simulink library "Decoders_Lib"  (Simulink 8.7)
settings: Solver=ode45  StartTime=0.0  StopTime=10.0  RelTol=1e-3
libraries: Computer_Library x17, commutil2 x5
(part 1 of 2)
settings Model: Creator=uzivatel  LastModifiedBy=Jozko Mrkvicka

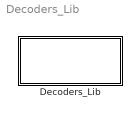
== system Decoders_Lib ==
  Decoders_Lib : Subsystem

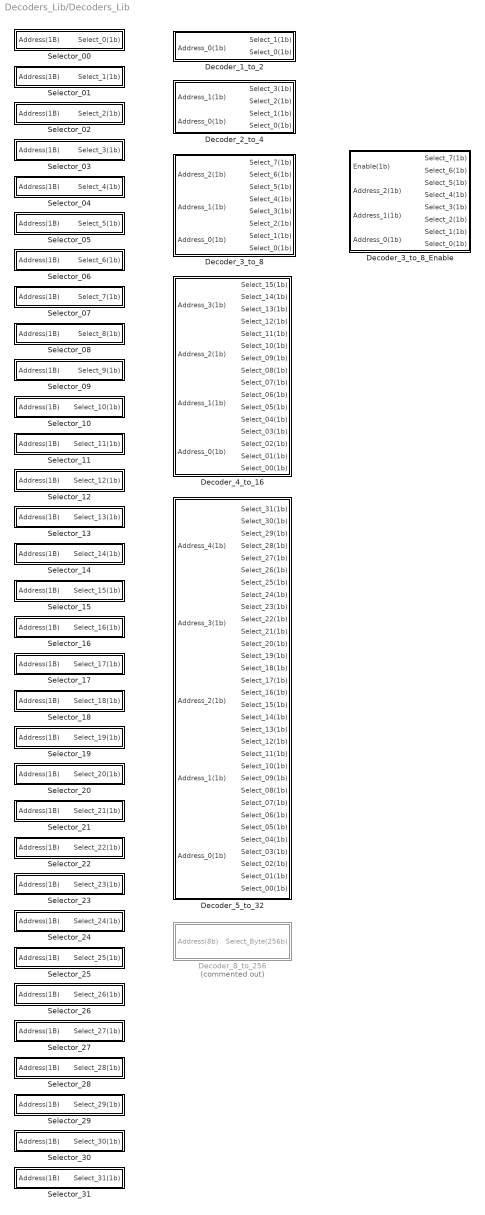
== system Decoders_Lib/Decoders_Lib ==
  Decoder_1_to_2 : Subsystem  TreatAsAtomicUnit=on
  Decoder_2_to_4 : Subsystem  TreatAsAtomicUnit=on
  Decoder_3_to_8 : Subsystem  TreatAsAtomicUnit=on
  Decoder_3_to_8_Enable : Subsystem  TreatAsAtomicUnit=on
  Decoder_4_to_16 : Subsystem  TreatAsAtomicUnit=on
  Decoder_5_to_32 : Subsystem  TreatAsAtomicUnit=on
  Decoder_8_to_256 : Subsystem  Commented=on
  Selector_00 : Subsystem
  Selector_01 : Subsystem
  Selector_02 : Subsystem
  Selector_03 : Subsystem
  Selector_04 : Subsystem
  Selector_05 : Subsystem
  Selector_06 : Subsystem
  Selector_07 : Subsystem
  Selector_08 : Subsystem
  Selector_09 : Subsystem
  Selector_10 : Subsystem
  Selector_11 : Subsystem
  Selector_12 : Subsystem
  Selector_13 : Subsystem
  Selector_14 : Subsystem
  Selector_15 : Subsystem
  Selector_16 : Subsystem
  Selector_17 : Subsystem
  Selector_18 : Subsystem
  Selector_19 : Subsystem
  Selector_20 : Subsystem
  Selector_21 : Subsystem
  Selector_22 : Subsystem
  Selector_23 : Subsystem
  Selector_24 : Subsystem
  Selector_25 : Subsystem
  Selector_26 : Subsystem
  Selector_27 : Subsystem
  Selector_28 : Subsystem
  Selector_29 : Subsystem
  Selector_30 : Subsystem
  Selector_31 : Subsystem

== system Decoders_Lib/Decoders_Lib/Decoder_1_to_2 ==
  Address_0(1b) : Inport
  Logical Operator23 : Logic  Operator=NOT  IconShape=distinctive  AllPortsSameDT=off  OutDataTypeStr=boolean
  Select_1(1b) : Outport
  Select_0(1b) : Outport  Port=2
  wires:
  Logical Operator23/1 -> Select_0(1b)/1
  Address_0(1b)/1 -> Logical Operator23/1, Select_1(1b)/1

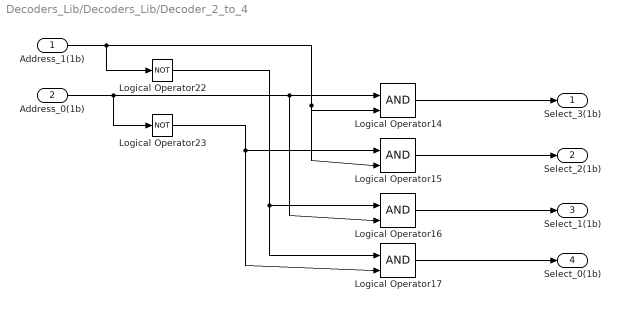
== system Decoders_Lib/Decoders_Lib/Decoder_2_to_4 ==
  Address_1(1b) : Inport
  Address_0(1b) : Inport  Port=2
  Logical Operator{14..17} (4 alike) : Logic  IconShape=distinctive  AllPortsSameDT=off  OutDataTypeStr=boolean
  Logical Operator22 : Logic  Operator=NOT  IconShape=distinctive  AllPortsSameDT=off  OutDataTypeStr=boolean
  Logical Operator23 : Logic  Operator=NOT  IconShape=distinctive  AllPortsSameDT=off  OutDataTypeStr=boolean
  Select_3(1b) : Outport
  Select_2(1b) : Outport  Port=2
  Select_1(1b) : Outport  Port=3
  Select_0(1b) : Outport  Port=4
  wires:
  Address_0(1b)/1 -> Logical Operator23/1, Logical Operator16/2, Logical Operator14/1
  Logical Operator22/1 -> Logical Operator16/1, Logical Operator17/1
  Logical Operator23/1 -> Logical Operator15/1, Logical Operator17/2
  Address_1(1b)/1 -> Logical Operator14/2, Logical Operator15/2, Logical Operator22/1
  Logical Operator17/1 -> Select_0(1b)/1
  Logical Operator16/1 -> Select_1(1b)/1
  Logical Operator15/1 -> Select_2(1b)/1
  Logical Operator14/1 -> Select_3(1b)/1

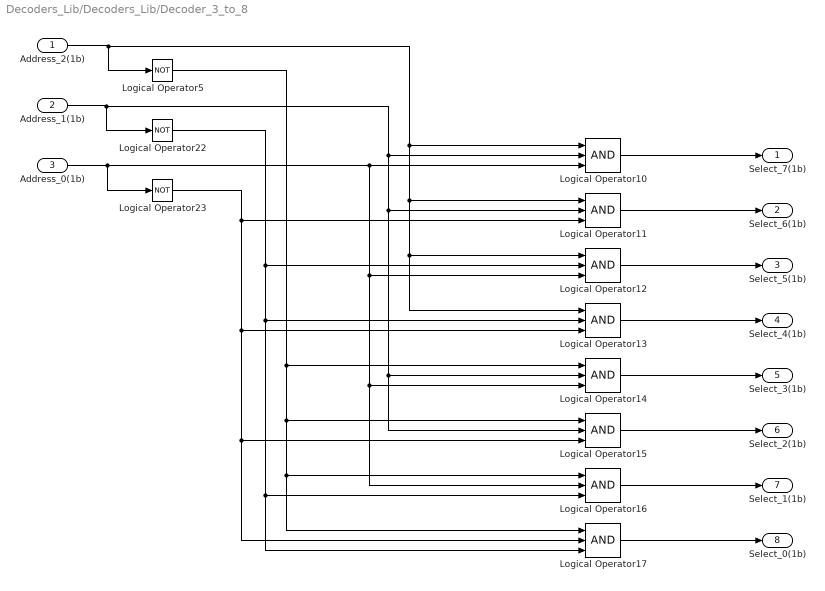
== system Decoders_Lib/Decoders_Lib/Decoder_3_to_8 ==
  "Address_2(1b) " : Inport
  Address_1(1b) : Inport  Port=2
  Address_0(1b) : Inport  Port=3
  Logical Operator{10..17} (8 alike) : Logic  Inputs=3  IconShape=distinctive  AllPortsSameDT=off  OutDataTypeStr=boolean
  Logical Operator22 : Logic  Operator=NOT  IconShape=distinctive  AllPortsSameDT=off  OutDataTypeStr=boolean
  Logical Operator23 : Logic  Operator=NOT  IconShape=distinctive  AllPortsSameDT=off  OutDataTypeStr=boolean
  Logical Operator5 : Logic  Operator=NOT  IconShape=distinctive  AllPortsSameDT=off  OutDataTypeStr=boolean
  Select_7(1b) : Outport
  Select_6(1b) : Outport  Port=2
  Select_5(1b) : Outport  Port=3
  Select_4(1b) : Outport  Port=4
  Select_3(1b) : Outport  Port=5
  Select_2(1b) : Outport  Port=6
  Select_1(1b) : Outport  Port=7
  Select_0(1b) : Outport  Port=8
  wires:
  Address_0(1b)/1 -> Logical Operator10/3, Logical Operator12/3, Logical Operator14/3, Logical Operator16/2, Logical Operator23/1
  Logical Operator22/1 -> Logical Operator12/2, Logical Operator13/2, Logical Operator16/3, Logical Operator17/3
  Logical Operator23/1 -> Logical Operator11/3, Logical Operator13/3, Logical Operator15/3, Logical Operator17/2
  Logical Operator5/1 -> Logical Operator14/1, Logical Operator15/1, Logical Operator16/1, Logical Operator17/1
  Address_1(1b)/1 -> Logical Operator10/2, Logical Operator11/2, Logical Operator14/2, Logical Operator15/2, Logical Operator22/1
  "Address_2(1b) "/1 -> Logical Operator10/1, Logical Operator11/1, Logical Operator12/1, Logical Operator13/1, Logical Operator5/1
  Logical Operator17/1 -> Select_0(1b)/1
  Logical Operator16/1 -> Select_1(1b)/1
  Logical Operator15/1 -> Select_2(1b)/1
  Logical Operator14/1 -> Select_3(1b)/1
  Logical Operator13/1 -> Select_4(1b)/1
  Logical Operator12/1 -> Select_5(1b)/1
  Logical Operator11/1 -> Select_6(1b)/1
  Logical Operator10/1 -> Select_7(1b)/1

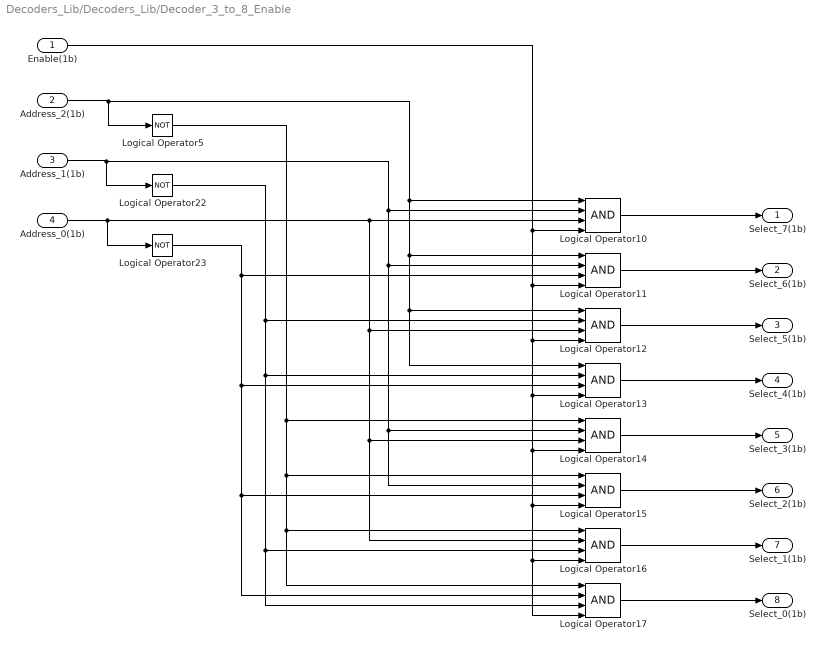
== system Decoders_Lib/Decoders_Lib/Decoder_3_to_8_Enable ==
  Enable(1b) : Inport
  "Address_2(1b) " : Inport  Port=2
  Address_1(1b) : Inport  Port=3
  Address_0(1b) : Inport  Port=4
  Logical Operator{10..17} (8 alike) : Logic  Inputs=4  IconShape=distinctive  AllPortsSameDT=off  OutDataTypeStr=boolean
  Logical Operator22 : Logic  Operator=NOT  IconShape=distinctive  AllPortsSameDT=off  OutDataTypeStr=boolean
  Logical Operator23 : Logic  Operator=NOT  IconShape=distinctive  AllPortsSameDT=off  OutDataTypeStr=boolean
  Logical Operator5 : Logic  Operator=NOT  IconShape=distinctive  AllPortsSameDT=off  OutDataTypeStr=boolean
  Select_7(1b) : Outport
  Select_6(1b) : Outport  Port=2
  Select_5(1b) : Outport  Port=3
  Select_4(1b) : Outport  Port=4
  Select_3(1b) : Outport  Port=5
  Select_2(1b) : Outport  Port=6
  Select_1(1b) : Outport  Port=7
  Select_0(1b) : Outport  Port=8
  wires:
  Address_0(1b)/1 -> Logical Operator10/3, Logical Operator12/3, Logical Operator14/3, Logical Operator16/2, Logical Operator23/1
  Logical Operator22/1 -> Logical Operator12/2, Logical Operator13/2, Logical Operator16/3, Logical Operator17/3
  Logical Operator23/1 -> Logical Operator11/3, Logical Operator13/3, Logical Operator15/3, Logical Operator17/2
  Logical Operator5/1 -> Logical Operator14/1, Logical Operator15/1, Logical Operator16/1, Logical Operator17/1
  Address_1(1b)/1 -> Logical Operator11/2, Logical Operator14/2, Logical Operator15/2, Logical Operator10/2, Logical Operator22/1
  "Address_2(1b) "/1 -> Logical Operator11/1, Logical Operator12/1, Logical Operator13/1, Logical Operator10/1, Logical Operator5/1
  Logical Operator17/1 -> Select_0(1b)/1
  Logical Operator16/1 -> Select_1(1b)/1
  Logical Operator15/1 -> Select_2(1b)/1
  Logical Operator14/1 -> Select_3(1b)/1
  Logical Operator13/1 -> Select_4(1b)/1
  Logical Operator12/1 -> Select_5(1b)/1
  Logical Operator11/1 -> Select_6(1b)/1
  Logical Operator10/1 -> Select_7(1b)/1
  Enable(1b)/1 -> Logical Operator10/4, Logical Operator11/4, Logical Operator12/4, Logical Operator14/4, Logical Operator15/4, Logical Operator16/4, Logical Operator17/4, Logical Operator13/4

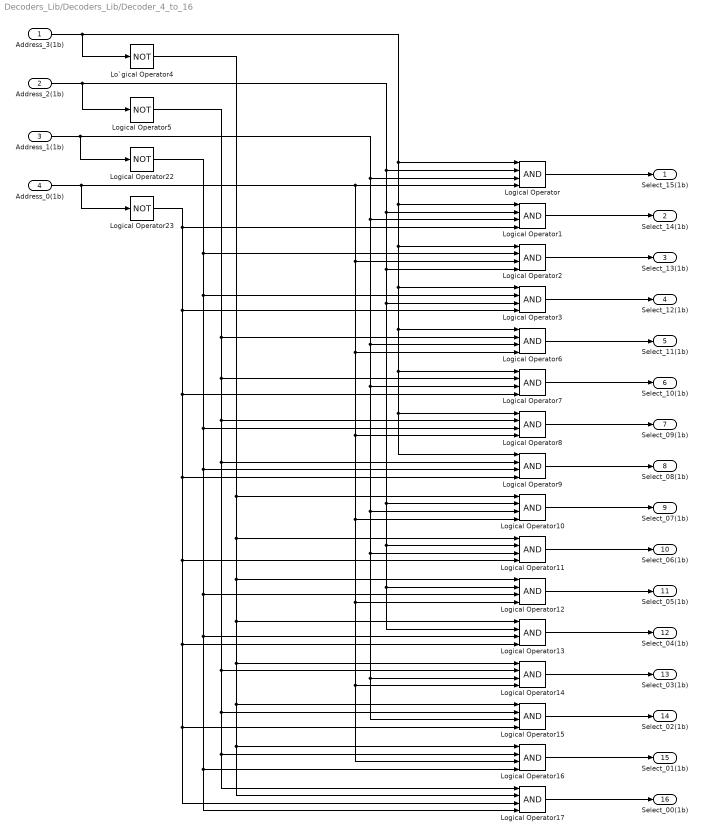
== system Decoders_Lib/Decoders_Lib/Decoder_4_to_16 ==
  Address_3(1b) : Inport
  "Address_2(1b) " : Inport  Port=2
  Address_1(1b) : Inport  Port=3
  Address_0(1b) : Inport  Port=4
  Lo`gical Operator4 : Logic  Operator=NOT  IconShape=distinctive  AllPortsSameDT=off  OutDataTypeStr=boolean
  Logical Operator{,1..3,6..17} (16 alike) : Logic  Inputs=4  IconShape=distinctive  AllPortsSameDT=off  OutDataTypeStr=boolean
  Logical Operator22 : Logic  Operator=NOT  IconShape=distinctive  AllPortsSameDT=off  OutDataTypeStr=boolean
  Logical Operator23 : Logic  Operator=NOT  IconShape=distinctive  AllPortsSameDT=off  OutDataTypeStr=boolean
  Logical Operator5 : Logic  Operator=NOT  IconShape=distinctive  AllPortsSameDT=off  OutDataTypeStr=boolean
  Select_15(1b) : Outport
  Select_14(1b) : Outport  Port=2
  Select_13(1b) : Outport  Port=3
  Select_12(1b) : Outport  Port=4
  Select_11(1b) : Outport  Port=5
  Select_10(1b) : Outport  Port=6
  Select_09(1b) : Outport  Port=7
  Select_08(1b) : Outport  Port=8
  Select_07(1b) : Outport  Port=9
  Select_06(1b) : Outport  Port=10
  Select_05(1b) : Outport  Port=11
  Select_04(1b) : Outport  Port=12
  Select_03(1b) : Outport  Port=13
  Select_02(1b) : Outport  Port=14
  Select_01(1b) : Outport  Port=15
  Select_00(1b) : Outport  Port=16
  wires:
  Logical Operator22/1 -> Logical Operator2/2, Logical Operator3/2, Logical Operator8/3, Logical Operator9/3, Logical Operator12/3, Logical Operator13/3, Logical Operator16/4, Logical Operator17/4
  Address_0(1b)/1 -> Logical Operator/4, Logical Operator2/3, Logical Operator6/4, Logical Operator8/4, Logical Operator10/4, Logical Operator12/4, Logical Operator14/4, Logical Operator16/3, Logical Operator23/1
  Logical Operator23/1 -> Logical Operator1/4, Logical Operator3/4, Logical Operator7/4, Logical Operator9/4, Logical Operator11/4, Logical Operator13/4, Logical Operator15/4, Logical Operator17/3
  Logical Operator5/1 -> Logical Operator6/2, Logical Operator7/2, Logical Operator8/2, Logical Operator9/2, Logical Operator14/2, Logical Operator15/2, Logical Operator16/2, Logical Operator17/1
  Address_3(1b)/1 -> Lo`gical Operator4/1, Logical Operator2/1, Logical Operator3/1, Logical Operator6/1, Logical Operator7/1, Logical Operator8/1, Logical Operator9/1, Logical Operator1/1, Logical Operator/1
  Address_1(1b)/1 -> Logical Operator22/1, Logical Operator/3, Logical Operator1/3, Logical Operator6/3, Logical Operator7/3, Logical Operator10/3, Logical Operator11/3, Logical Operator14/3, Logical Operator15/3
  "Address_2(1b) "/1 -> Logical Operator/2, Logical Operator1/2, Logical Operator2/4, Logical Operator3/3, Logical Operator10/2, Logical Operator11/2, Logical Operator12/2, Logical Operator13/2, Logical Operator5/1
  Lo`gical Operator4/1 -> Logical Operator10/1, Logical Operator11/1, Logical Operator12/1, Logical Operator13/1, Logical Operator14/1, Logical Operator15/1, Logical Operator16/1, Logical Operator17/2
  Logical Operator17/1 -> Select_00(1b)/1
  Logical Operator16/1 -> Select_01(1b)/1
  Logical Operator15/1 -> Select_02(1b)/1
  Logical Operator14/1 -> Select_03(1b)/1
  Logical Operator13/1 -> Select_04(1b)/1
  Logical Operator12/1 -> Select_05(1b)/1
  Logical Operator11/1 -> Select_06(1b)/1
  Logical Operator10/1 -> Select_07(1b)/1
  Logical Operator9/1 -> Select_08(1b)/1
  Logical Operator8/1 -> Select_09(1b)/1
  Logical Operator7/1 -> Select_10(1b)/1
  Logical Operator6/1 -> Select_11(1b)/1
  Logical Operator1/1 -> Select_14(1b)/1
  Logical Operator2/1 -> Select_13(1b)/1
  Logical Operator3/1 -> Select_12(1b)/1
  Logical Operator/1 -> Select_15(1b)/1

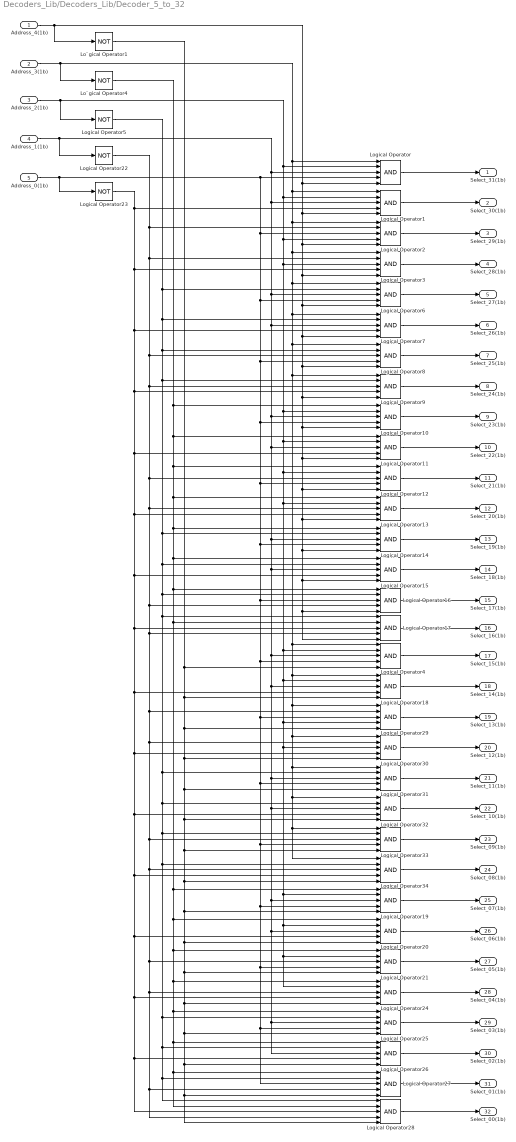
== system Decoders_Lib/Decoders_Lib/Decoder_5_to_32 ==
  Address_4(1b) : Inport
  Address_3(1b) : Inport  Port=2
  "Address_2(1b) " : Inport  Port=3
  Address_1(1b) : Inport  Port=4
  Address_0(1b) : Inport  Port=5
  Lo`gical Operator1 : Logic  Operator=NOT  IconShape=distinctive  AllPortsSameDT=off  OutDataTypeStr=boolean
  Lo`gical Operator4 : Logic  Operator=NOT  IconShape=distinctive  AllPortsSameDT=off  OutDataTypeStr=boolean
  Logical Operator{,1..4,6..21,24..34} (32 alike) : Logic  Inputs=5  IconShape=distinctive  AllPortsSameDT=off  OutDataTypeStr=boolean
  Logical Operator22 : Logic  Operator=NOT  IconShape=distinctive  AllPortsSameDT=off  OutDataTypeStr=boolean
  Logical Operator23 : Logic  Operator=NOT  IconShape=distinctive  AllPortsSameDT=off  OutDataTypeStr=boolean
  Logical Operator5 : Logic  Operator=NOT  IconShape=distinctive  AllPortsSameDT=off  OutDataTypeStr=boolean
  Select_31(1b) : Outport
  Select_30(1b) : Outport  Port=2
  Select_29(1b) : Outport  Port=3
  Select_28(1b) : Outport  Port=4
  Select_27(1b) : Outport  Port=5
  Select_26(1b) : Outport  Port=6
  Select_25(1b) : Outport  Port=7
  Select_24(1b) : Outport  Port=8
  Select_23(1b) : Outport  Port=9
  Select_22(1b) : Outport  Port=10
  Select_21(1b) : Outport  Port=11
  Select_20(1b) : Outport  Port=12
  Select_19(1b) : Outport  Port=13
  Select_18(1b) : Outport  Port=14
  Select_17(1b) : Outport  Port=15
  Select_16(1b) : Outport  Port=16
  Select_15(1b) : Outport  Port=17
  Select_14(1b) : Outport  Port=18
  Select_13(1b) : Outport  Port=19
  Select_12(1b) : Outport  Port=20
  Select_11(1b) : Outport  Port=21
  Select_10(1b) : Outport  Port=22
  Select_09(1b) : Outport  Port=23
  Select_08(1b) : Outport  Port=24
  Select_07(1b) : Outport  Port=25
  Select_06(1b) : Outport  Port=26
  Select_05(1b) : Outport  Port=27
  Select_04(1b) : Outport  Port=28
  Select_03(1b) : Outport  Port=29
  Select_02(1b) : Outport  Port=30
  Select_01(1b) : Outport  Port=31
  Select_00(1b) : Outport  Port=32
  wires:
  Logical Operator17/1 -> Select_16(1b)/1
  Logical Operator16/1 -> Select_17(1b)/1
  Logical Operator15/1 -> Select_18(1b)/1
  Logical Operator14/1 -> Select_19(1b)/1
  Logical Operator13/1 -> Select_20(1b)/1
  Logical Operator12/1 -> Select_21(1b)/1
  Logical Operator11/1 -> Select_22(1b)/1
  Logical Operator10/1 -> Select_23(1b)/1
  Logical Operator9/1 -> Select_24(1b)/1
  Logical Operator8/1 -> Select_25(1b)/1
  Logical Operator7/1 -> Select_26(1b)/1
  Logical Operator6/1 -> Select_27(1b)/1
  Logical Operator1/1 -> Select_30(1b)/1
  Logical Operator2/1 -> Select_29(1b)/1
  Logical Operator3/1 -> Select_28(1b)/1
  Logical Operator/1 -> Select_31(1b)/1
  Logical Operator22/1 -> Logical Operator8/3, Logical Operator9/3, Logical Operator12/3, Logical Operator13/3, Logical Operator16/4, Logical Operator29/2, Logical Operator30/2, Logical Operator33/3, Logical Operator34/3, Logical Operator21/3, Logical Operator24/3, Logical Operator27/4, Logical Operator28/4, Logical Operator17/4, Logical Operator3/2, Logical Operator2/2
  Address_0(1b)/1 -> Logical Operator/4, Logical Operator2/3, Logical Operator6/4, Logical Operator8/4, Logical Operator10/4, Logical Operator12/4, Logical Operator14/4, Logical Operator16/3, Logical Operator4/4, Logical Operator29/3, Logical Operator31/4, Logical Operator33/4, Logical Operator19/4, Logical Operator21/4, Logical Operator25/4, Logical Operator27/3, Logical Operator23/1
  Logical Operator23/1 -> Logical Operator1/4, Logical Operator3/4, Logical Operator7/4, Logical Operator9/4, Logical Operator11/4, Logical Operator13/4, Logical Operator15/4, Logical Operator18/4, Logical Operator30/4, Logical Operator32/4, Logical Operator34/4, Logical Operator20/4, Logical Operator24/4, Logical Operator26/4, Logical Operator28/3, Logical Operator17/3
  Logical Operator5/1 -> Logical Operator31/2, Logical Operator32/2, Logical Operator33/2, Logical Operator34/2, Logical Operator25/2, Logical Operator26/2, Logical Operator27/2, Logical Operator28/1, Logical Operator17/1, Logical Operator16/2, Logical Operator15/2, Logical Operator14/2, Logical Operator9/2, Logical Operator8/2, Logical Operator7/2, Logical Operator6/2
  Address_3(1b)/1 -> Lo`gical Operator4/1, Logical Operator2/1, Logical Operator3/1, Logical Operator6/1, Logical Operator7/1, Logical Operator8/1, Logical Operator4/1, Logical Operator18/1, Logical Operator29/1, Logical Operator30/1, Logical Operator31/1, Logical Operator32/1, Logical Operator33/1, Logical Operator34/1, Logical Operator9/1, Logical Operator1/1, Logical Operator/1
  Address_1(1b)/1 -> Logical Operator22/1, Logical Operator1/3, Logical Operator6/3, Logical Operator7/3, Logical Operator10/3, Logical Operator11/3, Logical Operator14/3, Logical Operator4/3, Logical Operator18/3, Logical Operator31/3, Logical Operator32/3, Logical Operator19/3, Logical Operator20/3, Logical Operator25/3, Logical Operator26/3, Logical Operator15/3, Logical Operator/3
  "Address_2(1b) "/1 -> Logical Operator2/4, Logical Operator3/3, Logical Operator4/2, Logical Operator18/2, Logical Operator29/4, Logical Operator30/3, Logical Operator19/2, Logical Operator20/2, Logical Operator21/2, Logical Operator24/2, Logical Operator13/2, Logical Operator12/2, Logical Operator11/2, Logical Operator10/2, Logical Operator1/2, Logical Operator/2, Logical Operator5/1
  Lo`gical Operator4/1 -> Logical Operator19/1, Logical Operator20/1, Logical Operator21/1, Logical Operator24/1, Logical Operator25/1, Logical Operator26/1, Logical Operator27/1, Logical Operator28/2, Logical Operator17/2, Logical Operator16/1, Logical Operator15/1, Logical Operator14/1, Logical Operator13/1, Logical Operator12/1, Logical Operator11/1, Logical Operator10/1
  Logical Operator28/1 -> Select_00(1b)/1
  Logical Operator27/1 -> Select_01(1b)/1
  Logical Operator26/1 -> Select_02(1b)/1
  Logical Operator25/1 -> Select_03(1b)/1
  Logical Operator24/1 -> Select_04(1b)/1
  Logical Operator21/1 -> Select_05(1b)/1
  Logical Operator20/1 -> Select_06(1b)/1
  Logical Operator19/1 -> Select_07(1b)/1
  Logical Operator34/1 -> Select_08(1b)/1
  Logical Operator33/1 -> Select_09(1b)/1
  Logical Operator32/1 -> Select_10(1b)/1
  Logical Operator31/1 -> Select_11(1b)/1
  Logical Operator18/1 -> Select_14(1b)/1
  Logical Operator29/1 -> Select_13(1b)/1
  Logical Operator30/1 -> Select_12(1b)/1
  Logical Operator4/1 -> Select_15(1b)/1
  Lo`gical Operator1/1 -> Logical Operator4/5, Logical Operator18/5, Logical Operator29/5, Logical Operator30/5, Logical Operator31/5, Logical Operator32/5, Logical Operator33/5, Logical Operator34/5, Logical Operator19/5, Logical Operator20/5, Logical Operator21/5, Logical Operator24/5, Logical Operator25/5, Logical Operator26/5, Logical Operator27/5, Logical Operator28/5
  Address_4(1b)/1 -> Lo`gical Operator1/1, Logical Operator/5, Logical Operator1/5, Logical Operator2/5, Logical Operator3/5, Logical Operator6/5, Logical Operator7/5, Logical Operator8/5, Logical Operator9/5, Logical Operator10/5, Logical Operator11/5, Logical Operator12/5, Logical Operator13/5, Logical Operator14/5, Logical Operator15/5, Logical Operator16/5, Logical Operator17/5

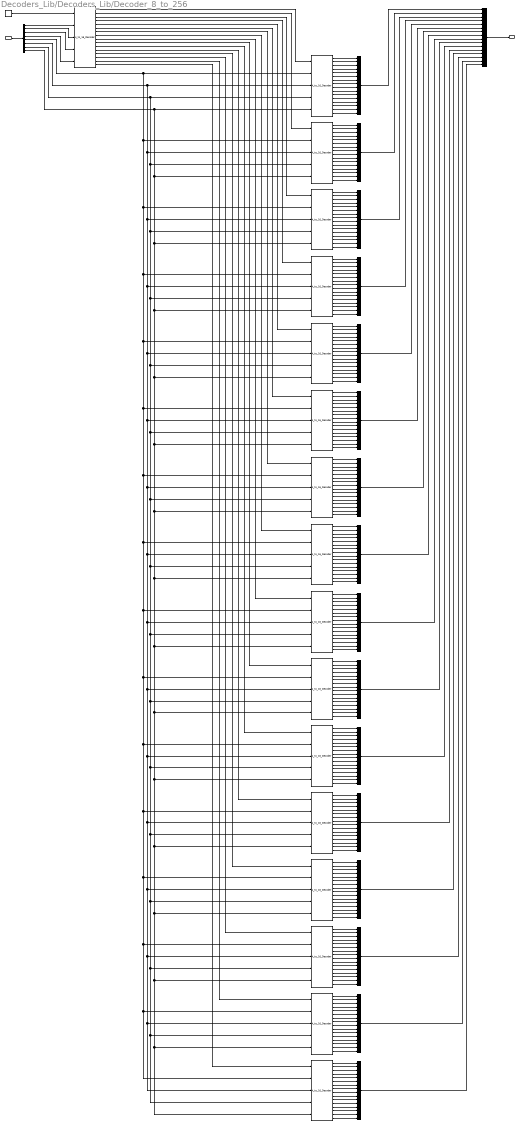
== system Decoders_Lib/Decoders_Lib/Decoder_8_to_256 ==
  Address(8b) : Inport
  4_to_16_Decoder{,1..16} (17 alike) : Computer_Library/4_to_16_Decoder
  Demux : Demux  Outputs=8
  Enable : Constant
  Mux{,1..16} (17 alike) : Mux  Inputs=16
  Select_Byte(256b) : Outport
  wires:
  Mux/1 -> Select_Byte(256b)/1
  Address(8b)/1 -> Demux/1
  Mux2/1 -> Mux/2
  Mux3/1 -> Mux/3
  Mux4/1 -> Mux/4
  Mux5/1 -> Mux/5
  Mux6/1 -> Mux/6
  Mux7/1 -> Mux/7
  Mux8/1 -> Mux/8
  Mux9/1 -> Mux/9
  Mux10/1 -> Mux/10
  Mux11/1 -> Mux/11
  Mux12/1 -> Mux/12
  Mux13/1 -> Mux/13
  Mux14/1 -> Mux/14
  Mux15/1 -> Mux/15
  Mux16/1 -> Mux/16
  Mux1/1 -> Mux/1
  4_to_16_Decoder16/16 -> Mux16/16
  4_to_16_Decoder16/15 -> Mux16/15
  4_to_16_Decoder16/14 -> Mux16/14
  4_to_16_Decoder16/13 -> Mux16/13
  4_to_16_Decoder16/12 -> Mux16/12
  4_to_16_Decoder16/11 -> Mux16/11
  4_to_16_Decoder16/10 -> Mux16/10
  4_to_16_Decoder16/9 -> Mux16/9
  4_to_16_Decoder16/8 -> Mux16/8
  4_to_16_Decoder16/7 -> Mux16/7
  4_to_16_Decoder16/6 -> Mux16/6
  4_to_16_Decoder16/5 -> Mux16/5
  4_to_16_Decoder16/4 -> Mux16/4
  4_to_16_Decoder16/3 -> Mux16/3
  4_to_16_Decoder16/2 -> Mux16/2
  4_to_16_Decoder16/1 -> Mux16/1
  4_to_16_Decoder15/16 -> Mux15/16
  4_to_16_Decoder15/15 -> Mux15/15
  4_to_16_Decoder15/14 -> Mux15/14
  4_to_16_Decoder15/13 -> Mux15/13
  4_to_16_Decoder15/12 -> Mux15/12
  4_to_16_Decoder15/11 -> Mux15/11
  4_to_16_Decoder15/10 -> Mux15/10
  4_to_16_Decoder15/9 -> Mux15/9
  4_to_16_Decoder15/8 -> Mux15/8
  4_to_16_Decoder15/7 -> Mux15/7
  4_to_16_Decoder15/6 -> Mux15/6
  4_to_16_Decoder15/5 -> Mux15/5
  4_to_16_Decoder15/4 -> Mux15/4
  4_to_16_Decoder15/3 -> Mux15/3
  4_to_16_Decoder15/2 -> Mux15/2
  4_to_16_Decoder15/1 -> Mux15/1
  4_to_16_Decoder14/16 -> Mux14/16
  4_to_16_Decoder14/15 -> Mux14/15
  4_to_16_Decoder14/14 -> Mux14/14
  4_to_16_Decoder14/13 -> Mux14/13
  4_to_16_Decoder14/12 -> Mux14/12
  4_to_16_Decoder14/11 -> Mux14/11
  4_to_16_Decoder14/10 -> Mux14/10
  4_to_16_Decoder14/9 -> Mux14/9
  4_to_16_Decoder14/8 -> Mux14/8
  4_to_16_Decoder14/7 -> Mux14/7
  4_to_16_Decoder14/6 -> Mux14/6
  4_to_16_Decoder14/5 -> Mux14/5
  4_to_16_Decoder14/4 -> Mux14/4
  4_to_16_Decoder14/3 -> Mux14/3
  4_to_16_Decoder14/2 -> Mux14/2
  4_to_16_Decoder14/1 -> Mux14/1
  4_to_16_Decoder13/16 -> Mux13/16
  4_to_16_Decoder13/15 -> Mux13/15
  4_to_16_Decoder13/14 -> Mux13/14
  4_to_16_Decoder13/13 -> Mux13/13
  4_to_16_Decoder13/12 -> Mux13/12
  4_to_16_Decoder13/11 -> Mux13/11
  4_to_16_Decoder13/10 -> Mux13/10
  4_to_16_Decoder13/9 -> Mux13/9
  4_to_16_Decoder13/8 -> Mux13/8
  4_to_16_Decoder13/7 -> Mux13/7
  4_to_16_Decoder13/6 -> Mux13/6
  4_to_16_Decoder13/5 -> Mux13/5
  4_to_16_Decoder13/4 -> Mux13/4
  4_to_16_Decoder13/3 -> Mux13/3
  4_to_16_Decoder13/2 -> Mux13/2
  4_to_16_Decoder13/1 -> Mux13/1
  4_to_16_Decoder12/16 -> Mux12/16
  4_to_16_Decoder12/15 -> Mux12/15
  4_to_16_Decoder12/14 -> Mux12/14
  4_to_16_Decoder12/13 -> Mux12/13
  4_to_16_Decoder12/12 -> Mux12/12
  4_to_16_Decoder12/11 -> Mux12/11
  4_to_16_Decoder12/10 -> Mux12/10
  4_to_16_Decoder12/9 -> Mux12/9
  4_to_16_Decoder12/8 -> Mux12/8
  4_to_16_Decoder12/7 -> Mux12/7
  4_to_16_Decoder12/6 -> Mux12/6
  4_to_16_Decoder12/5 -> Mux12/5
  4_to_16_Decoder12/4 -> Mux12/4
  4_to_16_Decoder12/3 -> Mux12/3
  4_to_16_Decoder12/2 -> Mux12/2
  4_to_16_Decoder12/1 -> Mux12/1
  4_to_16_Decoder11/16 -> Mux11/16
  4_to_16_Decoder11/15 -> Mux11/15
  4_to_16_Decoder11/14 -> Mux11/14
  4_to_16_Decoder11/13 -> Mux11/13
  4_to_16_Decoder11/12 -> Mux11/12
  4_to_16_Decoder11/11 -> Mux11/11
  4_to_16_Decoder11/10 -> Mux11/10
  4_to_16_Decoder11/9 -> Mux11/9
  4_to_16_Decoder11/8 -> Mux11/8
  4_to_16_Decoder11/7 -> Mux11/7
  4_to_16_Decoder11/6 -> Mux11/6
  4_to_16_Decoder11/5 -> Mux11/5
  4_to_16_Decoder11/4 -> Mux11/4
  4_to_16_Decoder11/3 -> Mux11/3
  4_to_16_Decoder11/2 -> Mux11/2
  4_to_16_Decoder11/1 -> Mux11/1
  4_to_16_Decoder10/16 -> Mux10/16
  4_to_16_Decoder10/15 -> Mux10/15
  4_to_16_Decoder10/14 -> Mux10/14
  4_to_16_Decoder10/13 -> Mux10/13
  4_to_16_Decoder10/12 -> Mux10/12
  4_to_16_Decoder10/11 -> Mux10/11
  4_to_16_Decoder10/10 -> Mux10/10
  4_to_16_Decoder10/9 -> Mux10/9
  4_to_16_Decoder10/8 -> Mux10/8
  4_to_16_Decoder10/7 -> Mux10/7
  4_to_16_Decoder10/6 -> Mux10/6
  4_to_16_Decoder10/5 -> Mux10/5
  4_to_16_Decoder10/4 -> Mux10/4
  4_to_16_Decoder10/3 -> Mux10/3
  4_to_16_Decoder10/2 -> Mux10/2
  4_to_16_Decoder10/1 -> Mux10/1
  4_to_16_Decoder9/16 -> Mux9/16
  4_to_16_Decoder9/15 -> Mux9/15
  4_to_16_Decoder9/14 -> Mux9/14
  4_to_16_Decoder9/13 -> Mux9/13
  4_to_16_Decoder9/12 -> Mux9/12
  4_to_16_Decoder9/11 -> Mux9/11
  4_to_16_Decoder9/10 -> Mux9/10
  4_to_16_Decoder9/9 -> Mux9/9
  4_to_16_Decoder9/8 -> Mux9/8
  4_to_16_Decoder9/7 -> Mux9/7
  4_to_16_Decoder9/6 -> Mux9/6
  4_to_16_Decoder9/5 -> Mux9/5
  4_to_16_Decoder9/4 -> Mux9/4
  4_to_16_Decoder9/3 -> Mux9/3
  4_to_16_Decoder9/2 -> Mux9/2
  4_to_16_Decoder9/1 -> Mux9/1
  4_to_16_Decoder8/16 -> Mux8/16
  4_to_16_Decoder8/15 -> Mux8/15
  4_to_16_Decoder8/14 -> Mux8/14
  4_to_16_Decoder8/13 -> Mux8/13
  4_to_16_Decoder8/12 -> Mux8/12
  4_to_16_Decoder8/11 -> Mux8/11
  4_to_16_Decoder8/10 -> Mux8/10
  4_to_16_Decoder8/9 -> Mux8/9
  4_to_16_Decoder8/8 -> Mux8/8
  4_to_16_Decoder8/7 -> Mux8/7
  4_to_16_Decoder8/6 -> Mux8/6
  4_to_16_Decoder8/5 -> Mux8/5
  4_to_16_Decoder8/4 -> Mux8/4
  4_to_16_Decoder8/3 -> Mux8/3
  4_to_16_Decoder8/2 -> Mux8/2
  4_to_16_Decoder8/1 -> Mux8/1
  4_to_16_Decoder7/16 -> Mux7/16
  4_to_16_Decoder7/15 -> Mux7/15
  4_to_16_Decoder7/14 -> Mux7/14
  4_to_16_Decoder7/13 -> Mux7/13
  4_to_16_Decoder7/12 -> Mux7/12
  4_to_16_Decoder7/11 -> Mux7/11
  4_to_16_Decoder7/10 -> Mux7/10
  4_to_16_Decoder7/9 -> Mux7/9
  4_to_16_Decoder7/8 -> Mux7/8
  4_to_16_Decoder7/7 -> Mux7/7
  4_to_16_Decoder7/6 -> Mux7/6
  4_to_16_Decoder7/5 -> Mux7/5
  4_to_16_Decoder7/4 -> Mux7/4
  4_to_16_Decoder7/3 -> Mux7/3
  4_to_16_Decoder7/2 -> Mux7/2
  4_to_16_Decoder7/1 -> Mux7/1
  4_to_16_Decoder6/16 -> Mux6/16
  4_to_16_Decoder6/15 -> Mux6/15
  4_to_16_Decoder6/14 -> Mux6/14
  4_to_16_Decoder6/13 -> Mux6/13
  4_to_16_Decoder6/12 -> Mux6/12
  4_to_16_Decoder6/11 -> Mux6/11
  4_to_16_Decoder6/10 -> Mux6/10
  4_to_16_Decoder6/9 -> Mux6/9
  4_to_16_Decoder6/8 -> Mux6/8
  4_to_16_Decoder6/7 -> Mux6/7
  4_to_16_Decoder6/6 -> Mux6/6
  4_to_16_Decoder6/5 -> Mux6/5
  4_to_16_Decoder6/4 -> Mux6/4
  4_to_16_Decoder6/3 -> Mux6/3
  4_to_16_Decoder6/2 -> Mux6/2
  4_to_16_Decoder6/1 -> Mux6/1
  4_to_16_Decoder5/16 -> Mux5/16
  4_to_16_Decoder5/15 -> Mux5/15
  4_to_16_Decoder5/14 -> Mux5/14
  4_to_16_Decoder5/13 -> Mux5/13
  4_to_16_Decoder5/12 -> Mux5/12
  4_to_16_Decoder5/11 -> Mux5/11
  4_to_16_Decoder5/10 -> Mux5/10
  4_to_16_Decoder5/9 -> Mux5/9
  4_to_16_Decoder5/8 -> Mux5/8
  4_to_16_Decoder5/7 -> Mux5/7
  4_to_16_Decoder5/6 -> Mux5/6
  4_to_16_Decoder5/5 -> Mux5/5
  4_to_16_Decoder5/4 -> Mux5/4
  4_to_16_Decoder5/3 -> Mux5/3
  4_to_16_Decoder5/2 -> Mux5/2
  4_to_16_Decoder5/1 -> Mux5/1
  4_to_16_Decoder4/16 -> Mux4/16
  4_to_16_Decoder4/15 -> Mux4/15
  4_to_16_Decoder4/14 -> Mux4/14
  4_to_16_Decoder4/13 -> Mux4/13
  4_to_16_Decoder4/12 -> Mux4/12
  4_to_16_Decoder4/11 -> Mux4/11
  4_to_16_Decoder4/10 -> Mux4/10
  4_to_16_Decoder4/9 -> Mux4/9
  4_to_16_Decoder4/8 -> Mux4/8
  4_to_16_Decoder4/7 -> Mux4/7
  4_to_16_Decoder4/6 -> Mux4/6
  4_to_16_Decoder4/5 -> Mux4/5
  4_to_16_Decoder4/4 -> Mux4/4
  4_to_16_Decoder4/3 -> Mux4/3
  4_to_16_Decoder4/2 -> Mux4/2
  4_to_16_Decoder4/1 -> Mux4/1
  4_to_16_Decoder3/16 -> Mux3/16
  4_to_16_Decoder3/15 -> Mux3/15
  4_to_16_Decoder3/14 -> Mux3/14
  4_to_16_Decoder3/13 -> Mux3/13
  4_to_16_Decoder3/12 -> Mux3/12
  4_to_16_Decoder3/11 -> Mux3/11
  4_to_16_Decoder3/10 -> Mux3/10
  4_to_16_Decoder3/9 -> Mux3/9
  4_to_16_Decoder3/8 -> Mux3/8
  4_to_16_Decoder3/7 -> Mux3/7
  4_to_16_Decoder3/6 -> Mux3/6
  4_to_16_Decoder3/5 -> Mux3/5
  4_to_16_Decoder3/4 -> Mux3/4
  4_to_16_Decoder3/3 -> Mux3/3
  4_to_16_Decoder3/2 -> Mux3/2
  4_to_16_Decoder3/1 -> Mux3/1
  4_to_16_Decoder2/16 -> Mux2/16
  4_to_16_Decoder2/15 -> Mux2/15
  4_to_16_Decoder2/14 -> Mux2/14
  4_to_16_Decoder2/13 -> Mux2/13
  4_to_16_Decoder2/12 -> Mux2/12
  4_to_16_Decoder2/11 -> Mux2/11
  4_to_16_Decoder2/10 -> Mux2/10
  4_to_16_Decoder2/9 -> Mux2/9
  4_to_16_Decoder2/8 -> Mux2/8
  4_to_16_Decoder2/7 -> Mux2/7
  4_to_16_Decoder2/6 -> Mux2/6
  4_to_16_Decoder2/5 -> Mux2/5
  4_to_16_Decoder2/4 -> Mux2/4
  4_to_16_Decoder2/3 -> Mux2/3
  4_to_16_Decoder2/2 -> Mux2/2
  4_to_16_Decoder2/1 -> Mux2/1
  4_to_16_Decoder1/16 -> Mux1/16
  4_to_16_Decoder1/15 -> Mux1/15
  4_to_16_Decoder1/14 -> Mux1/14
  4_to_16_Decoder1/13 -> Mux1/13
  4_to_16_Decoder1/12 -> Mux1/12
  4_to_16_Decoder1/11 -> Mux1/11
  4_to_16_Decoder1/10 -> Mux1/10
  4_to_16_Decoder1/9 -> Mux1/9
  4_to_16_Decoder1/8 -> Mux1/8
  4_to_16_Decoder1/7 -> Mux1/7
  4_to_16_Decoder1/6 -> Mux1/6
  4_to_16_Decoder1/5 -> Mux1/5
  4_to_16_Decoder1/4 -> Mux1/4
  4_to_16_Decoder1/3 -> Mux1/3
  4_to_16_Decoder1/2 -> Mux1/2
  4_to_16_Decoder1/1 -> Mux1/1
  Enable/1 -> 4_to_16_Decoder/1
  4_to_16_Decoder/16 -> 4_to_16_Decoder16/1
  4_to_16_Decoder/15 -> 4_to_16_Decoder15/1
  4_to_16_Decoder/14 -> 4_to_16_Decoder14/1
  4_to_16_Decoder/13 -> 4_to_16_Decoder13/1
  4_to_16_Decoder/12 -> 4_to_16_Decoder12/1
  4_to_16_Decoder/11 -> 4_to_16_Decoder11/1
  4_to_16_Decoder/10 -> 4_to_16_Decoder10/1
  4_to_16_Decoder/9 -> 4_to_16_Decoder9/1
  4_to_16_Decoder/8 -> 4_to_16_Decoder8/1
  4_to_16_Decoder/7 -> 4_to_16_Decoder7/1
  4_to_16_Decoder/6 -> 4_to_16_Decoder6/1
  4_to_16_Decoder/5 -> 4_to_16_Decoder5/1
  4_to_16_Decoder/4 -> 4_to_16_Decoder4/1
  4_to_16_Decoder/3 -> 4_to_16_Decoder3/1
  4_to_16_Decoder/2 -> 4_to_16_Decoder2/1
  4_to_16_Decoder/1 -> 4_to_16_Decoder1/1
  Demux/8 -> 4_to_16_Decoder15/5, 4_to_16_Decoder16/5, 4_to_16_Decoder14/5, 4_to_16_Decoder13/5, 4_to_16_Decoder12/5, 4_to_16_Decoder11/5, 4_to_16_Decoder10/5, 4_to_16_Decoder9/5, 4_to_16_Decoder8/5, 4_to_16_Decoder7/5, 4_to_16_Decoder6/5, 4_to_16_Decoder5/5, 4_to_16_Decoder4/5, 4_to_16_Decoder3/5, 4_to_16_Decoder2/5, 4_to_16_Decoder1/5
  Demux/7 -> 4_to_16_Decoder15/4, 4_to_16_Decoder16/4, 4_to_16_Decoder14/4, 4_to_16_Decoder13/4, 4_to_16_Decoder12/4, 4_to_16_Decoder11/4, 4_to_16_Decoder10/4, 4_to_16_Decoder9/4, 4_to_16_Decoder8/4, 4_to_16_Decoder7/4, 4_to_16_Decoder6/4, 4_to_16_Decoder5/4, 4_to_16_Decoder4/4, 4_to_16_Decoder3/4, 4_to_16_Decoder2/4, 4_to_16_Decoder1/4
  Demux/6 -> 4_to_16_Decoder15/3, 4_to_16_Decoder16/3, 4_to_16_Decoder14/3, 4_to_16_Decoder13/3, 4_to_16_Decoder12/3, 4_to_16_Decoder11/3, 4_to_16_Decoder10/3, 4_to_16_Decoder9/3, 4_to_16_Decoder8/3, 4_to_16_Decoder7/3, 4_to_16_Decoder6/3, 4_to_16_Decoder5/3, 4_to_16_Decoder4/3, 4_to_16_Decoder3/3, 4_to_16_Decoder2/3, 4_to_16_Decoder1/3
  Demux/5 -> 4_to_16_Decoder15/2, 4_to_16_Decoder16/2, 4_to_16_Decoder14/2, 4_to_16_Decoder13/2, 4_to_16_Decoder12/2, 4_to_16_Decoder11/2, 4_to_16_Decoder10/2, 4_to_16_Decoder9/2, 4_to_16_Decoder8/2, 4_to_16_Decoder7/2, 4_to_16_Decoder6/2, 4_to_16_Decoder5/2, 4_to_16_Decoder4/2, 4_to_16_Decoder3/2, 4_to_16_Decoder2/2, 4_to_16_Decoder1/2
  Demux/4 -> 4_to_16_Decoder/5
  Demux/3 -> 4_to_16_Decoder/4
  Demux/2 -> 4_to_16_Decoder/3
  Demux/1 -> 4_to_16_Decoder/2

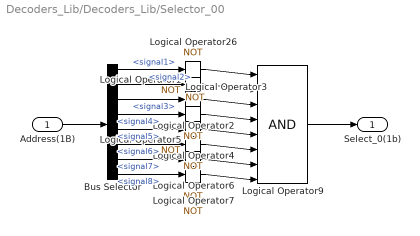
== system Decoders_Lib/Decoders_Lib/Selector_00 ==
  Address(1B) : Inport
  Bus Selector : BusSelector  OutputSignals=signal1,signal2,signal3,signal4,signal5,signal6,signal7,signal8
  Logical Operator{1..7,26} (8 alike) : Logic  Operator=NOT  Inputs=1  IconShape=distinctive  AllPortsSameDT=off  OutDataTypeStr=boolean
  Logical Operator9 : Logic  Inputs=8  IconShape=distinctive  AllPortsSameDT=off  OutDataTypeStr=boolean
  Select_0(1b) : Outport
  wires:
  Address(1B)/1 -> Bus Selector/1
  Logical Operator26/1 -> Logical Operator9/1
  Bus Selector/1 -> Logical Operator26/1  "<signal1>"
  Logical Operator9/1 -> Select_0(1b)/1
  Logical Operator1/1 -> Logical Operator9/2
  Bus Selector/2 -> Logical Operator1/1  "<signal2>"
  Logical Operator2/1 -> Logical Operator9/3
  Bus Selector/3 -> Logical Operator2/1  "<signal3>"
  Logical Operator3/1 -> Logical Operator9/4
  Bus Selector/4 -> Logical Operator3/1  "<signal4>"
  Logical Operator4/1 -> Logical Operator9/5
  Bus Selector/5 -> Logical Operator4/1  "<signal5>"
  Logical Operator5/1 -> Logical Operator9/6
  Bus Selector/6 -> Logical Operator5/1  "<signal6>"
  Logical Operator6/1 -> Logical Operator9/7
  Bus Selector/7 -> Logical Operator6/1  "<signal7>"
  Logical Operator7/1 -> Logical Operator9/8
  Bus Selector/8 -> Logical Operator7/1  "<signal8>"

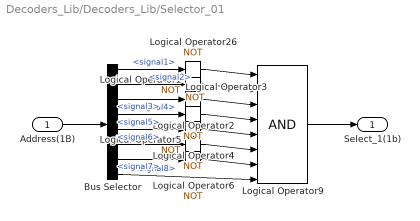
== system Decoders_Lib/Decoders_Lib/Selector_01 ==
  Address(1B) : Inport
  Bus Selector : BusSelector  OutputSignals=signal1,signal2,signal3,signal4,signal5,signal6,signal7,signal8
  Logical Operator{1..6,26} (7 alike) : Logic  Operator=NOT  Inputs=1  IconShape=distinctive  AllPortsSameDT=off  OutDataTypeStr=boolean
  Logical Operator9 : Logic  Inputs=8  IconShape=distinctive  AllPortsSameDT=off  OutDataTypeStr=boolean
  Select_1(1b) : Outport
  wires:
  Bus Selector/8 -> Logical Operator9/8  "<signal8>"
  Bus Selector/7 -> Logical Operator6/1  "<signal7>"
  Logical Operator6/1 -> Logical Operator9/7
  Bus Selector/6 -> Logical Operator5/1  "<signal6>"
  Logical Operator5/1 -> Logical Operator9/6
  Bus Selector/5 -> Logical Operator4/1  "<signal5>"
  Logical Operator4/1 -> Logical Operator9/5
  Bus Selector/4 -> Logical Operator3/1  "<signal4>"
  Logical Operator3/1 -> Logical Operator9/4
  Bus Selector/3 -> Logical Operator2/1  "<signal3>"
  Logical Operator2/1 -> Logical Operator9/3
  Bus Selector/2 -> Logical Operator1/1  "<signal2>"
  Logical Operator1/1 -> Logical Operator9/2
  Logical Operator9/1 -> Select_1(1b)/1
  Bus Selector/1 -> Logical Operator26/1  "<signal1>"
  Logical Operator26/1 -> Logical Operator9/1
  Address(1B)/1 -> Bus Selector/1

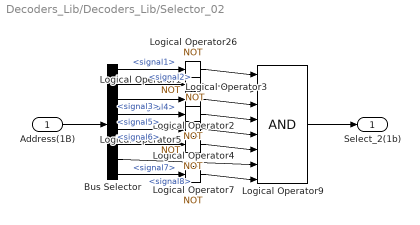
== system Decoders_Lib/Decoders_Lib/Selector_02 ==
  Address(1B) : Inport
  Bus Selector : BusSelector  OutputSignals=signal1,signal2,signal3,signal4,signal5,signal6,signal7,signal8
  Logical Operator{1..5,7,26} (7 alike) : Logic  Operator=NOT  Inputs=1  IconShape=distinctive  AllPortsSameDT=off  OutDataTypeStr=boolean
  Logical Operator9 : Logic  Inputs=8  IconShape=distinctive  AllPortsSameDT=off  OutDataTypeStr=boolean
  Select_2(1b) : Outport
  wires:
  Bus Selector/8 -> Logical Operator7/1  "<signal8>"
  Logical Operator7/1 -> Logical Operator9/8
  Bus Selector/7 -> Logical Operator9/7  "<signal7>"
  Bus Selector/6 -> Logical Operator5/1  "<signal6>"
  Logical Operator5/1 -> Logical Operator9/6
  Bus Selector/5 -> Logical Operator4/1  "<signal5>"
  Logical Operator4/1 -> Logical Operator9/5
  Bus Selector/4 -> Logical Operator3/1  "<signal4>"
  Logical Operator3/1 -> Logical Operator9/4
  Bus Selector/3 -> Logical Operator2/1  "<signal3>"
  Logical Operator2/1 -> Logical Operator9/3
  Bus Selector/2 -> Logical Operator1/1  "<signal2>"
  Logical Operator1/1 -> Logical Operator9/2
  Logical Operator9/1 -> Select_2(1b)/1
  Bus Selector/1 -> Logical Operator26/1  "<signal1>"
  Logical Operator26/1 -> Logical Operator9/1
  Address(1B)/1 -> Bus Selector/1

== system Decoders_Lib/Decoders_Lib/Selector_03 ==
  Address(1B) : Inport
  Bus Selector : BusSelector  OutputSignals=signal1,signal2,signal3,signal4,signal5,signal6,signal7,signal8
  Logical Operator{1..5,26} (6 alike) : Logic  Operator=NOT  Inputs=1  IconShape=distinctive  AllPortsSameDT=off  OutDataTypeStr=boolean
  Logical Operator9 : Logic  Inputs=8  IconShape=distinctive  AllPortsSameDT=off  OutDataTypeStr=boolean
  Select_3(1b) : Outport
  wires:
  Bus Selector/8 -> Logical Operator9/8  "<signal8>"
  Bus Selector/7 -> Logical Operator9/7  "<signal7>"
  Bus Selector/6 -> Logical Operator5/1  "<signal6>"
  Logical Operator5/1 -> Logical Operator9/6
  Bus Selector/5 -> Logical Operator4/1  "<signal5>"
  Logical Operator4/1 -> Logical Operator9/5
  Bus Selector/4 -> Logical Operator3/1  "<signal4>"
  Logical Operator3/1 -> Logical Operator9/4
  Bus Selector/3 -> Logical Operator2/1  "<signal3>"
  Logical Operator2/1 -> Logical Operator9/3
  Bus Selector/2 -> Logical Operator1/1  "<signal2>"
  Logical Operator1/1 -> Logical Operator9/2
  Logical Operator9/1 -> Select_3(1b)/1
  Bus Selector/1 -> Logical Operator26/1  "<signal1>"
  Logical Operator26/1 -> Logical Operator9/1
  Address(1B)/1 -> Bus Selector/1

== system Decoders_Lib/Decoders_Lib/Selector_04 ==
  Address(1B) : Inport
  Bus Selector : BusSelector  OutputSignals=signal1,signal2,signal3,signal4,signal5,signal6,signal7,signal8
  Logical Operator{1..4,6..7,26} (7 alike) : Logic  Operator=NOT  Inputs=1  IconShape=distinctive  AllPortsSameDT=off  OutDataTypeStr=boolean
  Logical Operator9 : Logic  Inputs=8  IconShape=distinctive  AllPortsSameDT=off  OutDataTypeStr=boolean
  Select_4(1b) : Outport
  wires:
  Bus Selector/8 -> Logical Operator7/1  "<signal8>"
  Logical Operator7/1 -> Logical Operator9/8
  Bus Selector/7 -> Logical Operator6/1  "<signal7>"
  Logical Operator6/1 -> Logical Operator9/7
  Bus Selector/6 -> Logical Operator9/6  "<signal6>"
  Bus Selector/5 -> Logical Operator4/1  "<signal5>"
  Logical Operator4/1 -> Logical Operator9/5
  Bus Selector/4 -> Logical Operator3/1  "<signal4>"
  Logical Operator3/1 -> Logical Operator9/4
  Bus Selector/3 -> Logical Operator2/1  "<signal3>"
  Logical Operator2/1 -> Logical Operator9/3
  Bus Selector/2 -> Logical Operator1/1  "<signal2>"
  Logical Operator1/1 -> Logical Operator9/2
  Logical Operator9/1 -> Select_4(1b)/1
  Bus Selector/1 -> Logical Operator26/1  "<signal1>"
  Logical Operator26/1 -> Logical Operator9/1
  Address(1B)/1 -> Bus Selector/1

== system Decoders_Lib/Decoders_Lib/Selector_05 ==
  Address(1B) : Inport
  Bus Selector : BusSelector  OutputSignals=signal1,signal2,signal3,signal4,signal5,signal6,signal7,signal8
  Logical Operator{1..4,6,26} (6 alike) : Logic  Operator=NOT  Inputs=1  IconShape=distinctive  AllPortsSameDT=off  OutDataTypeStr=boolean
  Logical Operator9 : Logic  Inputs=8  IconShape=distinctive  AllPortsSameDT=off  OutDataTypeStr=boolean
  Select_5(1b) : Outport
  wires:
  Bus Selector/8 -> Logical Operator9/8  "<signal8>"
  Bus Selector/7 -> Logical Operator6/1  "<signal7>"
  Logical Operator6/1 -> Logical Operator9/7
  Bus Selector/6 -> Logical Operator9/6  "<signal6>"
  Bus Selector/5 -> Logical Operator4/1  "<signal5>"
  Logical Operator4/1 -> Logical Operator9/5
  Bus Selector/4 -> Logical Operator3/1  "<signal4>"
  Logical Operator3/1 -> Logical Operator9/4
  Bus Selector/3 -> Logical Operator2/1  "<signal3>"
  Logical Operator2/1 -> Logical Operator9/3
  Bus Selector/2 -> Logical Operator1/1  "<signal2>"
  Logical Operator1/1 -> Logical Operator9/2
  Logical Operator9/1 -> Select_5(1b)/1
  Bus Selector/1 -> Logical Operator26/1  "<signal1>"
  Logical Operator26/1 -> Logical Operator9/1
  Address(1B)/1 -> Bus Selector/1

== system Decoders_Lib/Decoders_Lib/Selector_06 ==
  Address(1B) : Inport
  Demux : Demux  Outputs=8
  Integer to Bit Converter9 : commutil2/Integer to Bit Converter  nbits=8  signedInputValues=Unsigned  bitOrder=MSB first  outDtype=boolean
  Logical Operator{1..4,7,26} (6 alike) : Logic  Operator=NOT  Inputs=1  IconShape=distinctive  AllPortsSameDT=off  OutDataTypeStr=boolean
  Logical Operator9 : Logic  Inputs=8  IconShape=distinctive  AllPortsSameDT=off  OutDataTypeStr=boolean
  Select_6(1b) : Outport
  wires:
  Demux/8 -> Logical Operator7/1
  Logical Operator7/1 -> Logical Operator9/8
  Demux/7 -> Logical Operator9/7
  Demux/6 -> Logical Operator9/6
  Demux/5 -> Logical Operator4/1
  Logical Operator4/1 -> Logical Operator9/5
  Demux/4 -> Logical Operator3/1
  Logical Operator3/1 -> Logical Operator9/4
  Demux/3 -> Logical Operator2/1
  Logical Operator2/1 -> Logical Operator9/3
  Demux/2 -> Logical Operator1/1
  Logical Operator1/1 -> Logical Operator9/2
  Logical Operator9/1 -> Select_6(1b)/1
  Demux/1 -> Logical Operator26/1
  Logical Operator26/1 -> Logical Operator9/1
  Address(1B)/1 -> Integer to Bit Converter9/1
  Integer to Bit Converter9/1 -> Demux/1

== system Decoders_Lib/Decoders_Lib/Selector_07 ==
  Address(1B) : Inport
  Bus Selector : BusSelector  OutputSignals=signal1,signal2,signal3,signal4,signal5,signal6,signal7,signal8
  Logical Operator{1..4,26} (5 alike) : Logic  Operator=NOT  Inputs=1  IconShape=distinctive  AllPortsSameDT=off  OutDataTypeStr=boolean
  Logical Operator9 : Logic  Inputs=8  IconShape=distinctive  AllPortsSameDT=off  OutDataTypeStr=boolean
  Select_7(1b) : Outport
  wires:
  Bus Selector/8 -> Logical Operator9/8  "<signal8>"
  Bus Selector/7 -> Logical Operator9/7  "<signal7>"
  Bus Selector/6 -> Logical Operator9/6  "<signal6>"
  Bus Selector/5 -> Logical Operator4/1  "<signal5>"
  Logical Operator4/1 -> Logical Operator9/5
  Bus Selector/4 -> Logical Operator3/1  "<signal4>"
  Logical Operator3/1 -> Logical Operator9/4
  Bus Selector/3 -> Logical Operator2/1  "<signal3>"
  Logical Operator2/1 -> Logical Operator9/3
  Bus Selector/2 -> Logical Operator1/1  "<signal2>"
  Logical Operator1/1 -> Logical Operator9/2
  Logical Operator9/1 -> Select_7(1b)/1
  Bus Selector/1 -> Logical Operator26/1  "<signal1>"
  Logical Operator26/1 -> Logical Operator9/1
  Address(1B)/1 -> Bus Selector/1

== system Decoders_Lib/Decoders_Lib/Selector_08 ==
  Address(1B) : Inport
  Bus Selector : BusSelector  OutputSignals=signal1,signal2,signal3,signal4,signal5,signal6,signal7,signal8
  Logical Operator{1..3,5..7,26} (7 alike) : Logic  Operator=NOT  Inputs=1  IconShape=distinctive  AllPortsSameDT=off  OutDataTypeStr=boolean
  Logical Operator9 : Logic  Inputs=8  IconShape=distinctive  AllPortsSameDT=off  OutDataTypeStr=boolean
  Select_8(1b) : Outport
  wires:
  Bus Selector/8 -> Logical Operator7/1  "<signal8>"
  Logical Operator7/1 -> Logical Operator9/8
  Bus Selector/7 -> Logical Operator6/1  "<signal7>"
  Logical Operator6/1 -> Logical Operator9/7
  Bus Selector/6 -> Logical Operator5/1  "<signal6>"
  Logical Operator5/1 -> Logical Operator9/6
  Bus Selector/5 -> Logical Operator9/5  "<signal5>"
  Bus Selector/4 -> Logical Operator3/1  "<signal4>"
  Logical Operator3/1 -> Logical Operator9/4
  Bus Selector/3 -> Logical Operator2/1  "<signal3>"
  Logical Operator2/1 -> Logical Operator9/3
  Bus Selector/2 -> Logical Operator1/1  "<signal2>"
  Logical Operator1/1 -> Logical Operator9/2
  Logical Operator9/1 -> Select_8(1b)/1
  Bus Selector/1 -> Logical Operator26/1  "<signal1>"
  Logical Operator26/1 -> Logical Operator9/1
  Address(1B)/1 -> Bus Selector/1

== system Decoders_Lib/Decoders_Lib/Selector_09 ==
  Address(1B) : Inport
  Bus Selector : BusSelector  OutputSignals=signal1,signal2,signal3,signal4,signal5,signal6,signal7,signal8
  Logical Operator{1..3,5..6,26} (6 alike) : Logic  Operator=NOT  Inputs=1  IconShape=distinctive  AllPortsSameDT=off  OutDataTypeStr=boolean
  Logical Operator9 : Logic  Inputs=8  IconShape=distinctive  AllPortsSameDT=off  OutDataTypeStr=boolean
  Select_9(1b) : Outport
  wires:
  Bus Selector/8 -> Logical Operator9/8  "<signal8>"
  Bus Selector/7 -> Logical Operator6/1  "<signal7>"
  Logical Operator6/1 -> Logical Operator9/7
  Bus Selector/6 -> Logical Operator5/1  "<signal6>"
  Logical Operator5/1 -> Logical Operator9/6
  Bus Selector/5 -> Logical Operator9/5  "<signal5>"
  Bus Selector/4 -> Logical Operator3/1  "<signal4>"
  Logical Operator3/1 -> Logical Operator9/4
  Bus Selector/3 -> Logical Operator2/1  "<signal3>"
  Logical Operator2/1 -> Logical Operator9/3
  Bus Selector/2 -> Logical Operator1/1  "<signal2>"
  Logical Operator1/1 -> Logical Operator9/2
  Logical Operator9/1 -> Select_9(1b)/1
  Bus Selector/1 -> Logical Operator26/1  "<signal1>"
  Logical Operator26/1 -> Logical Operator9/1
  Address(1B)/1 -> Bus Selector/1

== system Decoders_Lib/Decoders_Lib/Selector_10 ==
  Address(1B) : Inport
  Bus Selector : BusSelector  OutputSignals=signal1,signal2,signal3,signal4,signal5,signal6,signal7,signal8
  Logical Operator{1..3,5,7,26} (6 alike) : Logic  Operator=NOT  Inputs=1  IconShape=distinctive  AllPortsSameDT=off  OutDataTypeStr=boolean
  Logical Operator9 : Logic  Inputs=8  IconShape=distinctive  AllPortsSameDT=off  OutDataTypeStr=boolean
  Select_10(1b) : Outport
  wires:
  Bus Selector/8 -> Logical Operator7/1  "<signal8>"
  Logical Operator7/1 -> Logical Operator9/8
  Bus Selector/7 -> Logical Operator9/7  "<signal7>"
  Bus Selector/6 -> Logical Operator5/1  "<signal6>"
  Logical Operator5/1 -> Logical Operator9/6
  Bus Selector/5 -> Logical Operator9/5  "<signal5>"
  Bus Selector/4 -> Logical Operator3/1  "<signal4>"
  Logical Operator3/1 -> Logical Operator9/4
  Bus Selector/3 -> Logical Operator2/1  "<signal3>"
  Logical Operator2/1 -> Logical Operator9/3
  Bus Selector/2 -> Logical Operator1/1  "<signal2>"
  Logical Operator1/1 -> Logical Operator9/2
  Logical Operator9/1 -> Select_10(1b)/1
  Bus Selector/1 -> Logical Operator26/1  "<signal1>"
  Logical Operator26/1 -> Logical Operator9/1
  Address(1B)/1 -> Bus Selector/1

== system Decoders_Lib/Decoders_Lib/Selector_11 ==
  Address(1B) : Inport
  Bus Selector : BusSelector  OutputSignals=signal1,signal2,signal3,signal4,signal5,signal6,signal7,signal8
  Logical Operator{1..3,5,26} (5 alike) : Logic  Operator=NOT  Inputs=1  IconShape=distinctive  AllPortsSameDT=off  OutDataTypeStr=boolean
  Logical Operator9 : Logic  Inputs=8  IconShape=distinctive  AllPortsSameDT=off  OutDataTypeStr=boolean
  Select_11(1b) : Outport
  wires:
  Bus Selector/8 -> Logical Operator9/8  "<signal8>"
  Bus Selector/7 -> Logical Operator9/7  "<signal7>"
  Bus Selector/6 -> Logical Operator5/1  "<signal6>"
  Logical Operator5/1 -> Logical Operator9/6
  Bus Selector/5 -> Logical Operator9/5  "<signal5>"
  Bus Selector/4 -> Logical Operator3/1  "<signal4>"
  Logical Operator3/1 -> Logical Operator9/4
  Bus Selector/3 -> Logical Operator2/1  "<signal3>"
  Logical Operator2/1 -> Logical Operator9/3
  Bus Selector/2 -> Logical Operator1/1  "<signal2>"
  Logical Operator1/1 -> Logical Operator9/2
  Logical Operator9/1 -> Select_11(1b)/1
  Bus Selector/1 -> Logical Operator26/1  "<signal1>"
  Logical Operator26/1 -> Logical Operator9/1
  Address(1B)/1 -> Bus Selector/1

== system Decoders_Lib/Decoders_Lib/Selector_12 ==
  Address(1B) : Inport
  Bus Selector : BusSelector  OutputSignals=signal1,signal2,signal3,signal4,signal5,signal6,signal7,signal8
  Logical Operator{1..3,6..7,26} (6 alike) : Logic  Operator=NOT  Inputs=1  IconShape=distinctive  AllPortsSameDT=off  OutDataTypeStr=boolean
  Logical Operator9 : Logic  Inputs=8  IconShape=distinctive  AllPortsSameDT=off  OutDataTypeStr=boolean
  Select_12(1b) : Outport
  wires:
  Bus Selector/8 -> Logical Operator7/1  "<signal8>"
  Logical Operator7/1 -> Logical Operator9/8
  Bus Selector/7 -> Logical Operator6/1  "<signal7>"
  Logical Operator6/1 -> Logical Operator9/7
  Bus Selector/6 -> Logical Operator9/6  "<signal6>"
  Bus Selector/5 -> Logical Operator9/5  "<signal5>"
  Bus Selector/4 -> Logical Operator3/1  "<signal4>"
  Logical Operator3/1 -> Logical Operator9/4
  Bus Selector/3 -> Logical Operator2/1  "<signal3>"
  Logical Operator2/1 -> Logical Operator9/3
  Bus Selector/2 -> Logical Operator1/1  "<signal2>"
  Logical Operator1/1 -> Logical Operator9/2
  Logical Operator9/1 -> Select_12(1b)/1
  Bus Selector/1 -> Logical Operator26/1  "<signal1>"
  Logical Operator26/1 -> Logical Operator9/1
  Address(1B)/1 -> Bus Selector/1

== system Decoders_Lib/Decoders_Lib/Selector_13 ==
  Address(1B) : Inport
  Bus Selector : BusSelector  OutputSignals=signal1,signal2,signal3,signal4,signal5,signal6,signal7,signal8
  Logical Operator{1..3,6,26} (5 alike) : Logic  Operator=NOT  Inputs=1  IconShape=distinctive  AllPortsSameDT=off  OutDataTypeStr=boolean
  Logical Operator9 : Logic  Inputs=8  IconShape=distinctive  AllPortsSameDT=off  OutDataTypeStr=boolean
  Select_13(1b) : Outport
  wires:
  Bus Selector/8 -> Logical Operator9/8  "<signal8>"
  Bus Selector/7 -> Logical Operator6/1  "<signal7>"
  Logical Operator6/1 -> Logical Operator9/7
  Bus Selector/6 -> Logical Operator9/6  "<signal6>"
  Bus Selector/5 -> Logical Operator9/5  "<signal5>"
  Bus Selector/4 -> Logical Operator3/1  "<signal4>"
  Logical Operator3/1 -> Logical Operator9/4
  Bus Selector/3 -> Logical Operator2/1  "<signal3>"
  Logical Operator2/1 -> Logical Operator9/3
  Bus Selector/2 -> Logical Operator1/1  "<signal2>"
  Logical Operator1/1 -> Logical Operator9/2
  Logical Operator9/1 -> Select_13(1b)/1
  Bus Selector/1 -> Logical Operator26/1  "<signal1>"
  Logical Operator26/1 -> Logical Operator9/1
  Address(1B)/1 -> Bus Selector/1

== system Decoders_Lib/Decoders_Lib/Selector_14 ==
  Address(1B) : Inport
  Bus Selector : BusSelector  OutputSignals=signal1,signal2,signal3,signal4,signal5,signal6,signal7,signal8
  Logical Operator{1..3,7,26} (5 alike) : Logic  Operator=NOT  Inputs=1  IconShape=distinctive  AllPortsSameDT=off  OutDataTypeStr=boolean
  Logical Operator9 : Logic  Inputs=8  IconShape=distinctive  AllPortsSameDT=off  OutDataTypeStr=boolean
  Select_14(1b) : Outport
  wires:
  Bus Selector/8 -> Logical Operator7/1  "<signal8>"
  Logical Operator7/1 -> Logical Operator9/8
  Bus Selector/7 -> Logical Operator9/7  "<signal7>"
  Bus Selector/6 -> Logical Operator9/6  "<signal6>"
  Bus Selector/5 -> Logical Operator9/5  "<signal5>"
  Bus Selector/4 -> Logical Operator3/1  "<signal4>"
  Logical Operator3/1 -> Logical Operator9/4
  Bus Selector/3 -> Logical Operator2/1  "<signal3>"
  Logical Operator2/1 -> Logical Operator9/3
  Bus Selector/2 -> Logical Operator1/1  "<signal2>"
  Logical Operator1/1 -> Logical Operator9/2
  Logical Operator9/1 -> Select_14(1b)/1
  Bus Selector/1 -> Logical Operator26/1  "<signal1>"
  Logical Operator26/1 -> Logical Operator9/1
  Address(1B)/1 -> Bus Selector/1

== system Decoders_Lib/Decoders_Lib/Selector_15 ==
  Address(1B) : Inport
  Bus Selector : BusSelector  OutputSignals=signal1,signal2,signal3,signal4,signal5,signal6,signal7,signal8
  Logical Operator{1..3,26} (4 alike) : Logic  Operator=NOT  Inputs=1  IconShape=distinctive  AllPortsSameDT=off  OutDataTypeStr=boolean
  Logical Operator9 : Logic  Inputs=8  IconShape=distinctive  AllPortsSameDT=off  OutDataTypeStr=boolean
  Select_15(1b) : Outport
  wires:
  Bus Selector/8 -> Logical Operator9/8  "<signal8>"
  Bus Selector/7 -> Logical Operator9/7  "<signal7>"
  Bus Selector/6 -> Logical Operator9/6  "<signal6>"
  Bus Selector/5 -> Logical Operator9/5  "<signal5>"
  Bus Selector/4 -> Logical Operator3/1  "<signal4>"
  Logical Operator3/1 -> Logical Operator9/4
  Bus Selector/3 -> Logical Operator2/1  "<signal3>"
  Logical Operator2/1 -> Logical Operator9/3
  Bus Selector/2 -> Logical Operator1/1  "<signal2>"
  Logical Operator1/1 -> Logical Operator9/2
  Logical Operator9/1 -> Select_15(1b)/1
  Bus Selector/1 -> Logical Operator26/1  "<signal1>"
  Logical Operator26/1 -> Logical Operator9/1
  Address(1B)/1 -> Bus Selector/1
